simulink model "fibonacci"  (R2020a)
settings: Solver=FixedStepDiscrete  StartTime=0.0  StopTime=6  FixedStep=T  RelTol=1e-3  EnableMultiTasking=on
settings Model: ExtModeTrigDuration=10000  Creator=mc218k  LastModifiedBy=mc218k
settings SolverCC: PositivePriorityOrder=on
settings DebuggingCC: ArithmeticOperatorsInVariantConditions=warning
settings SFSimCC: CustomCodeUndefinedFunction=UseInterfaceOnly
settings RTWCC: Description=QUARC Win64 Target  SystemTargetFile=quarc_win64.tlc  TemplateMakefile=quarc_default_tmf
settings STFCustomTargetCC: TargetPreCompLibLocation=C:\PROGRA~3\QUARC\lib\2019a\win64\release  TargetLangStandard=C99 (ISO)  ConcurrentExecutionCompliant=on  GRTInterface=on  SystemTargetFile=quarc_win64.tlc
settings GRTTargetCC: TargetPreCompLibLocation=C:\PROGRA~3\QUARC\lib\2019a\win64\release  ParMdlRefBuildCompliant=off  CompOptLevelCompliant=off  CombineOutputUpdateFcns=off  MatFileLogging=off  CPPClassGenCompliant=off  GRTInterface=on  UseToolchainInfoCompliant=off  ExtMode=on  ExtModeMexFile=quarc_comm

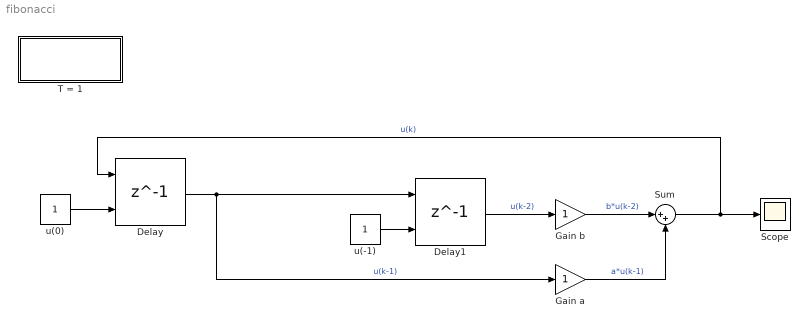
== system fibonacci ==
  Delay : Delay  DelayLength=1  InitialConditionSource=Input port
      settings: InputPortMap=u0,p4
  Delay1 : Delay  DelayLength=1  InitialConditionSource=Input port
      settings: InputPortMap=u0,p4
  Gain a : Gain
  Gain b : Gain
  Scope : Scope
  Sum : Sum  Inputs=|++
  T = 1 : Subsystem
      settings: OpenFcn=T=1;
  u(-1) : Constant
  u(0) : Constant
  wires:
  Delay/1 -> Delay1/1, Gain a/1  "u(k-1)"
  Delay1/1 -> Gain b/1  "u(k-2)"
  Sum/1 -> Delay/1, Scope/1  "u(k)"
  u(-1)/1 -> Delay1/2
  u(0)/1 -> Delay/2
  Gain a/1 -> Sum/2  "a*u(k-1)"
  Gain b/1 -> Sum/1  "b*u(k-2)"

== system fibonacci/T = 1 ==
